simulink model "SOC_Model"  (R2022b)
settings: Solver=VariableStepAuto  StartTime=0.0  StopTime=1  RelTol=1e-3
libraries: spsGroundLib x1, spsThreePhaseDynamicLoadLib x1, spsThreePhaseSeriesRLCBranchLib x1, spsThreePhaseSourceLib x1, spspowerguiLib x1
settings Model: Creator=Sajid Ali  LastModifiedBy=Sajid Ali

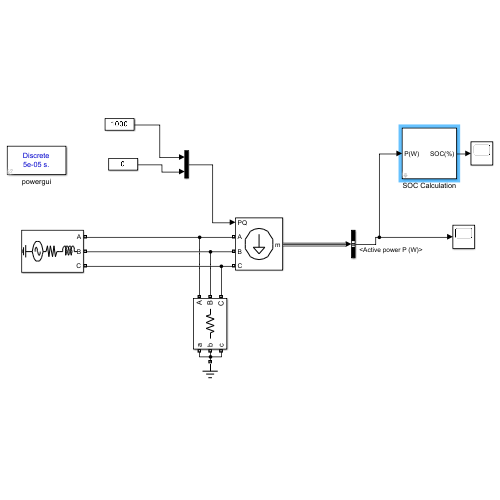
[thumbnail: Simulink's stored preview of the top-level diagram]
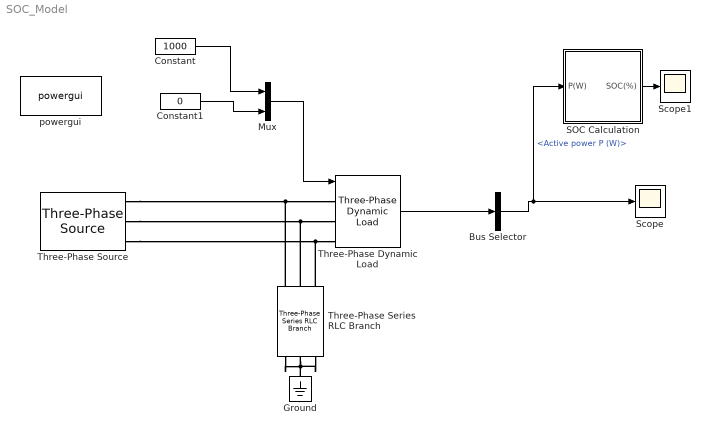
== system SOC_Model ==
  Bus Selector : BusSelector  OutputSignals=Active power P (W)
  Constant : Constant  Value=1000
  Constant1 : Constant  Value=0
  Ground : spsGroundLib/Ground  LConnTagsString=a
  Mux : Mux  Inputs=2
  SOC Calculation : Subsystem  mask{Erated=1, SOCinit=50}
      mask prompts: Erated "Battery Capacity (kWh)"; SOCinit "Initial State Of Charge (%)"
      mask DialogControl DescGroupVar Prompt: Model Description
      mask DialogControl DescTextVar Prompt: This subsystem Calculated the State Of Charge (SOC) by coulomb's counting method
      mask DialogControl ParameterGroupVar Prompt: System Characteristics
  Scope : Scope
  Scope1 : Scope
  Three-Phase Dynamic Load : spsThreePhaseDynamicLoadLib/Three-Phase Dynamic Load  NominalVoltage=[ 500e3 60 ]  ActiveReactivePowers=[50e6 25e6]  PositiveSequence=[0.994 -11.8]  ExternalControl=on  NpNq=[1.3 2]  TimeConstants="[0  0  0  0]"  MinimumVoltage=0.7  Tfilter=1e-4  LoadFlowParameters=[4,0,0,0,0]
      settings: LibrarySourceBlock=|
      | sps_lib/Passives/Three-Phase
      | Dynamic Load
  Three-Phase Series RLC Branch : spsThreePhaseSeriesRLCBranchLib/Three-Phase Series RLC Branch  LConnTagsString=A|B|C  RConnTagsString=A|B|C  BranchType=R  Resistance=1e9  Inductance=1e-3  Capacitance=1e-6  Measurements=None
  Three-Phase Source : spsThreePhaseSourceLib/Three-Phase Source  InternalConnection=Yg  VoltagePhases=off  Voltage=25e3  PhaseAngle=0  Voltage_phases=[25e3 25e3 25e3]/sqrt(3)  PhaseAngles_phases=[0 -120 +120]  Frequency=60  NonIdealSource=on  SpecifyImpedance=off  Resistance=0.8929  Inductance=16.58e-3  ShortCircuitLevel=100e6  BaseVoltage=25e3  XRratio=7  BusType=swing  Pref=10e3  Qref=0  Prefabc=[10e3, 10e3, 10e3]  Qrefabc=[0, 0, 0]  Qmin=-inf  Qmax=inf
  powergui : spspowerguiLib/powergui  Priority=1  SimulationMode=Discrete  SampleTime=50e-6  frequency=60  Iterations=50  frequencyindice=60  Pbase=100e6  ErrMax=1e-4  UnitsV=kV  UnitsW=MW  buscounter=0  FunctionMessages=off  echomessages=off  EnableUseOfTLC=off  CurrentSourceSwitches=off  DisableSnubberDevices=off  DisableRonSwitches=off  DisableVfSwitches=off  DisplayEquations=off  AutomaticDiscreteSolvers=off  SolverType=Tustin/Backward Euler (TBE)  Interpol=off  ExternalGateDelay=off  methode=off  Ts=100  x0status=blocks  SPID=on  SwTol=0  HookPort=off  NonlinearTolerance=1e-4  nMaxIteration=100  ContinueOnMaxIteration=off  RestoreLinks=warning  ResistiveCurrentMeasurement=off  Frange=[0:2:500]  Ylog=off  Xlog=on  ShowGrid=off  save=off  variable=ZData  structure=0  ZoomFFT=off  StartTime=0.0  cycles=1  DisplayStyle=1  fundamental=60  FreqAxis=off  MaxFrequency=1000  frequencyindicesteady=1  RmsSteady=1  display=off
  wires:
  Three-Phase Dynamic Load/1 -> Bus Selector/1
  Mux/1 -> Three-Phase Dynamic Load/1
  Constant/1 -> Mux/1
  Constant1/1 -> Mux/2
  Bus Selector/1 -> SOC Calculation/1(P(W)), Scope/1  "<Active power P (W)>"
  SOC Calculation/1(SOC(%)) -> Scope1/1
  connections:
  Three-Phase Source/RConn1 -- Three-Phase Series RLC Branch/LConn1 -- Three-Phase Dynamic Load/LConn1
  Three-Phase Source/RConn2 -- Three-Phase Series RLC Branch/LConn2 -- Three-Phase Dynamic Load/LConn2
  Three-Phase Source/RConn3 -- Three-Phase Series RLC Branch/LConn3 -- Three-Phase Dynamic Load/LConn3
  Ground/LConn1 -- Three-Phase Series RLC Branch/RConn3 -- Three-Phase Series RLC Branch/RConn1 -- Three-Phase Series RLC Branch/RConn2

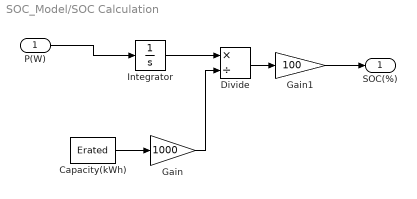
== system SOC_Model/SOC Calculation ==
  P(W) : Inport
  Capacity(kWh) : Constant  Value=Erated
  Divide : Product  Inputs=*/
  Gain : Gain  Gain=1000
  Gain1 : Gain  Gain=100
  Integrator : Integrator  InitialCondition=(SOCinit/100)*Erated*1000
  SOC(%) : Outport
  wires:
  P(W)/1 -> Integrator/1
  Integrator/1 -> Divide/1
  Capacity(kWh)/1 -> Gain/1
  Gain/1 -> Divide/2
  Divide/1 -> Gain1/1
  Gain1/1 -> SOC(%)/1
